simulink model "arduino_single_motor_IN1_IN2"  (R2021b)
settings: Solver=FixedStepAuto  StartTime=0.0  StopTime=inf  RelTol=1e-3
libraries: arduinolib x2, arduinosensorlib x1, simulink x1
settings Model: ExtModeTrigDuration=2  Creator=dbomb  LastModifiedBy=dbomb
settings OptimizationCC: EnhancedBackFolding=on  PassReuseOutputArgsAs=Individual arguments  ZeroExternalMemoryAtStartup=off  ZeroInternalMemoryAtStartup=off  MaxStackSize=64  OptimizeBlockOrder=speed  DifferentSizesBufferReuse=on  OptimizationCustomize=off  EfficientTunableParamExpr=on
settings DebuggingCC: ParameterTunabilityLossMsg=error
settings HardwareCC: ProdBitPerInt=16  ProdBitPerPointer=16  ProdBitPerSizeT=16  ProdBitPerPtrDiffT=16  ProdLargestAtomicFloat=None  ProdWordSize=8  ProdHWDeviceType=Atmel->AVR
settings SFSimCC: MATLABDynamicMemAlloc=off
settings RTWCC: Description=Embedded Coder  SystemTargetFile=ert.tlc  HardwareBoard=Arduino Mega 2560  TemplateMakefile=ert_default_tmf  Toolchain=Arduino AVR
settings CodeAppCC: ForceParamTrailComments=on  IgnoreCustomStorageClasses=off  OperatorAnnotations=on  SimulinkDataObjDesc=on  SFDataObjDesc=on  InsertBlockDesc=on
settings ERTTargetCC: SupportContinuousTime=on  SupportVariableSizeSignals=on  ExtModeTransport=3  ExtModeStaticAlloc=on  ExtModeStaticAllocSize=2048  ExtModeMexFile=ext_xcp  ExtModeIntrfLevel=Level2 - Open

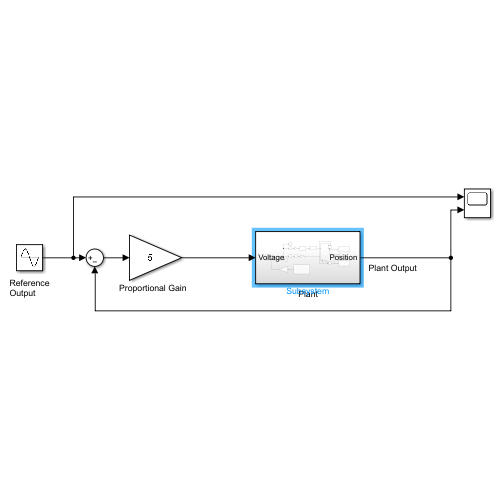
[thumbnail: Simulink's stored preview of the top-level diagram]
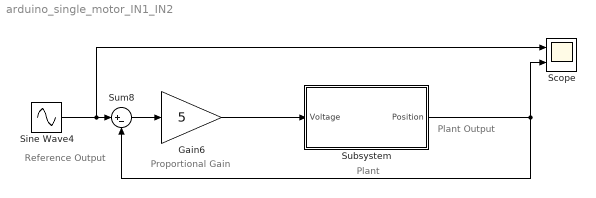
== system arduino_single_motor_IN1_IN2 ==
  note: Plant
  note: Proportional Gain
  note: Plant Output
  note: Reference
      | Output
  Gain6 : Gain  Gain=5
  Scope : Scope  NumInputPorts=2
  Sine Wave4 : Sin  Amplitude=25  Bias=25  Frequency=0.5  SampleTime=0
  Subsystem : Subsystem
  Sum8 : Sum  Inputs=|+-
  wires:
  Sine Wave4/1 -> Scope/1, Sum8/1
  Sum8/1 -> Gain6/1
  Subsystem/1(Position) -> Scope/2, Sum8/2
  Gain6/1 -> Subsystem/1(Voltage)

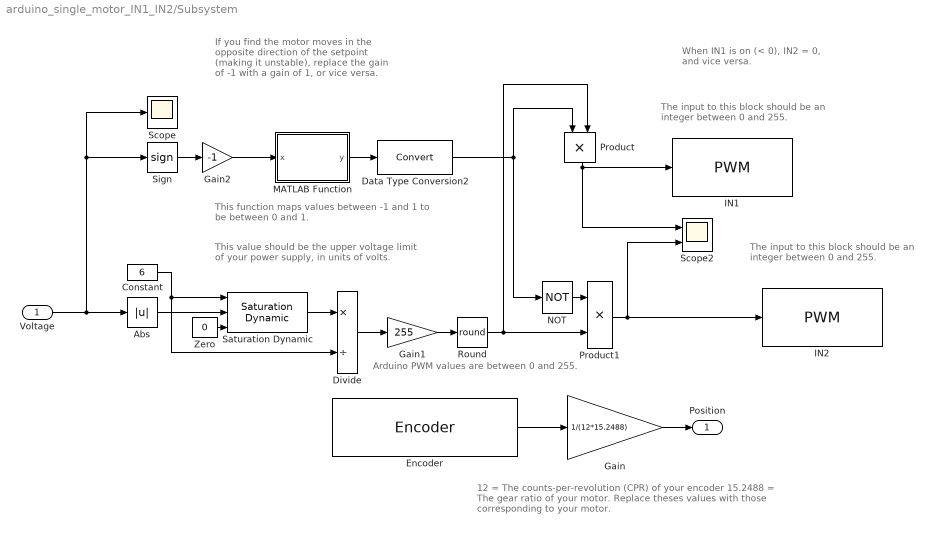
== system arduino_single_motor_IN1_IN2/Subsystem ==
  note: When IN1 is on (< 0), IN2 = 0, and vice versa.
  note: Arduino PWM values are between 0 and 255.
  note: This value should be the upper voltage
      | limit of your power supply, in units of volts.
  note: This function maps values between -1 and 1
      | to be between 0 and 1.
  note: 12 = The counts-per-revolution (CPR) of your encoder
      | 15.2488 = The gear ratio of your motor.
      | Replace theses values with those corresponding to your motor.
  note: If you find the motor moves in the opposite direction of the setpoint (making it unstable), replace the gain of -1 with a gain of 1, or vice versa.
  note: The input to this block should be
      | an integer between 0 and 255.
  note: The input to this block should be
      | an integer between 0 and 255.
  Voltage : Inport
  Abs : Abs
  Constant : Constant  Value=6
  Data Type Conversion2 : DataTypeConversion
  Divide : Product  Inputs=*/
  Encoder : arduinosensorlib/Encoder  InputA=2  InputB=3  Mode=No reset  SampleTime=-1
      settings: SourceProductBaseCode=ARDUINO
  Gain : Gain  Gain=1/(12*15.2488)
  Gain1 : Gain  Gain=255
  Gain2 : Gain  Gain=-1
  IN1 : arduinolib/PWM  pinNumber=9  frequencyType=Default  desiredFrequency=490.2  achievableFrequency=490.2
  IN2 : arduinolib/PWM  pinNumber=10  frequencyType=Default  desiredFrequency=490.2  achievableFrequency=490.2
  MATLAB Function : MATLAB Function  TreatAsAtomicUnit=on
  NOT : Logic  Operator=NOT  IconShape=distinctive  AllPortsSameDT=off  OutDataTypeStr=boolean
  Product : Product
  Product1 : Product
  Round : Rounding  Operator=round
  Saturation Dynamic : simulink/Discontinuities/Saturation Dynamic  OutMin=[]  OutMax=[]  OutDataTypeStr=Inherit: Same as second input  OutDataType=fixdt(1, 16)  OutScaling=2^-10  DoSatur=off
  Scope : Scope
  Scope2 : Scope  NumInputPorts=2
  Sign : Signum
  Zero : Constant  Value=0  OutDataTypeStr=Inherit: Inherit via back propagation
  Position : Outport
  wires:
  Gain2/1 -> MATLAB Function/1(x)
  Abs/1 -> Saturation Dynamic/2
  MATLAB Function/1(y) -> Data Type Conversion2/1
  Encoder/1 -> Gain/1
  Voltage/1 -> Sign/1, Scope/1, Abs/1
  Gain/1 -> Position/1
  Sign/1 -> Gain2/1
  Data Type Conversion2/1 -> Product/1, NOT/1
  Gain1/1 -> Round/1
  Product1/1 -> Scope2/2, IN2/1
  Product/1 -> IN1/1, Scope2/1
  NOT/1 -> Product1/1
  Constant/1 -> Saturation Dynamic/1, Divide/2
  Saturation Dynamic/1 -> Divide/1
  Divide/1 -> Gain1/1
  Zero/1 -> Saturation Dynamic/3
  Round/1 -> Product/2, Product1/2

== matlab function arduino_single_motor_IN1_IN2/Subsystem/MATLAB Function ==
  data: x input; y output
function y = fcn(x)
x = x*1;
y = 0.5*(x+1);
